simulink model "SIM_MDL"  (R2025b)
settings: Solver=ode4  StartTime=0.0  StopTime=5400  FixedStep=0.05  RelTol=1e-3
undefined symbols (not defined in the file): simData
settings Model: PauseTimes=600  Creator=antoniohernandez-rodiciomateos  LastModifiedBy=antoniohernandez-rodiciomateos

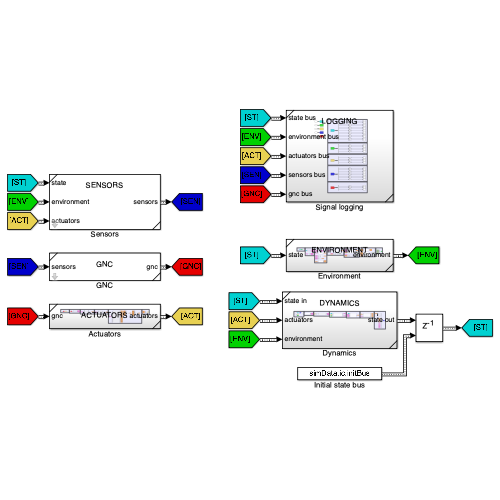
[thumbnail: Simulink's stored preview of the top-level diagram]
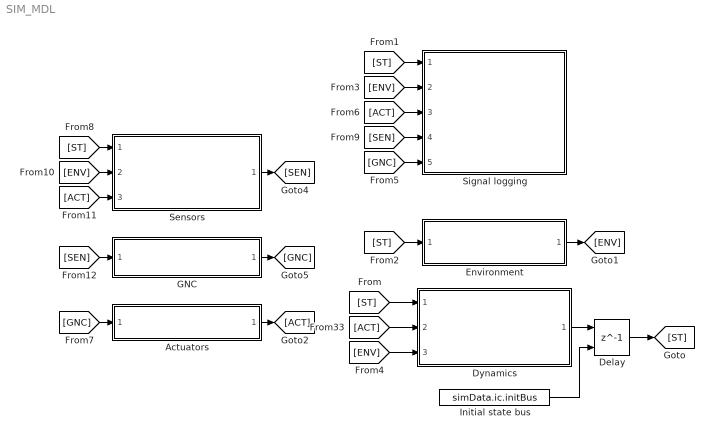
== system SIM_MDL ==
  Actuators : Subsystem  ReferencedSubsystem=ACTUATORS
  Delay : Delay  DelayLength=1  InitialConditionSource=Input port  InitialCondition=simData.ic.initBus
      settings: InputPortMap=u0,p4
  Dynamics : Subsystem  ReferencedSubsystem=DYNAMICS
  Environment : Subsystem  ReferencedSubsystem=ENVIRONMENT
  GNC : Subsystem  ReferencedSubsystem=GNC  initMode=simData.gnc.modes.initMode  omgBodSafeTH=simData.gnc.modes.omgBodSafeTH  omgRwDesaturationTH=simData.gnc.modes.omgRwDesaturationTH  omgRwDesaturationEndTH=simData.gnc.modes.omgRwDesaturationEndTH  omgRwMax=simData.rw.rwMaxOmg  targetAttEci=simData.gnc.gui.targetAttEci  fineNavMode=simData.gnc.nav.fineNavMode  desatK=simData.gnc.con.desatK  finePointKp=simData.gnc.con.finePointKp  finePointKd=simData.gnc.con.finePointKd  finePointKn=simData.gnc.con.finePointKn  mtqMagneticGain=simData.gnc.act.mtqMagneticGain  mtqResistance=simData.gnc.act.mtqResistance  mtqMaxVoltage=simData.gnc.act.mtqMaxVoltage  mtqMaxMagDip=simData.gnc.act.mtqMaxMagDip  mtqAllocationMatrix=simData.gnc.act.mtqAllocationMatrix  rwInertia=simData.gnc.act.rwInertia  rwMaxTorque=simData.gnc.act.rwMaxTorque  rwAllocationMatrix=simData.gnc.act.rwAllocationMatrix  magUpdateFreq=simData.mag.magUpdateFreq  refTimePosix=simData.cts.refTime  omgCelBod=simData.cts.omgCelBod  initGNCBus=simData.gnc.ic.initBus
  Initial state bus : Constant  Value=simData.ic.initBus  OutDataTypeStr=Bus: state_bus
  Sensors : Subsystem  ReferencedSubsystem=SENSORS  gyrUpdateFreq=simData.gyr.gyrUpdateFreq  gyrMeasLim=simData.gyr.gyrMeasLim  gyrARWperChannel=simData.gyr.gyrARWperChannel  gyrNoiseSeeds=simData.gyr.gyrNoiseSeeds  magUpdateFreq=simData.mag.magUpdateFreq  magMeasLim=simData.mag.magMeasLim  magNoisePerChannel=simData.mag.magNoisePerChannel  magNoiseSeeds=simData.mag.magNoiseSeeds  strUpdateFreq=simData.str.strUpdateFreq  strNoisePerChannel=simData.str.strNoisePerChannel  strBiasPerChannel=simData.str.strBias  strNoiseSeeds=simData.str.strNoiseSeeds  gnssUpdateFreq=simData.gnss.gnssUpdateFreq  gnssHorzAcc=simData.gnss.gnssHorzAcc  gnssVertAcc=simData.gnss.gnssVertAcc  gnssVelAcc=simData.gnss.gnssVelAcc  rweUpdateFreq=simData.rwe.rweUpdateFreq  simFixedStep=simData.sim.simTimeStep
  Signal logging : Subsystem  ReferencedSubsystem=LOGGING
  wires:
  Dynamics/1 -> Delay/1
  Delay/1 -> [ST]
  [ST] -> Dynamics/1
  Initial state bus/1 -> Delay/2
  [ST] -> Environment/1
  Environment/1 -> [ENV]
  [ENV] -> Dynamics/3
  [ACT] -> Dynamics/2
  Actuators/1 -> [ACT]
  [ST] -> Signal logging/1
  [ENV] -> Signal logging/2
  [GNC] -> Signal logging/5
  [ACT] -> Signal logging/3
  [GNC] -> Actuators/1
  [ST] -> Sensors/1
  Sensors/1 -> [SEN]
  [SEN] -> Signal logging/4
  [ENV] -> Sensors/2
  [ACT] -> Sensors/3
  GNC/1 -> [GNC]
  [SEN] -> GNC/1
